simulink model "RefModel_SystemIdentification"  (R2020a)
settings: Solver=ode1  StartTime=0.0  StopTime=inf  FixedStep=Ts_SystemIdentification.Ts_base  MaxStep=Ts  RelTol=1e-3
undefined symbols (not defined in the file or in its folder): SYS_IDENTIFICATION_PARAM
libraries: slctrlblks x4
settings Model: Creator=sl  LastModifiedBy=Administrator
settings DataIOCC: SaveOutput=off  SaveTime=off
settings OptimizationCC: DefaultParameterBehavior=Inlined  EnhancedBackFolding=on  PassReuseOutputArgsAs=Individual arguments  ZeroExternalMemoryAtStartup=off  ZeroInternalMemoryAtStartup=off  OptimizeBlockOrder=speed  DifferentSizesBufferReuse=on  OptimizationCustomize=off  EfficientTunableParamExpr=on
settings DebuggingCC: InheritedTsInSrcMsg=none  ParameterPrecisionLossMsg=none  ParameterTunabilityLossMsg=error  UnconnectedInputMsg=none  UnconnectedOutputMsg=none  UnconnectedLineMsg=none
settings HardwareCC: ProdBitPerPointer=32  ProdBitPerSizeT=32  ProdBitPerPtrDiffT=32  ProdLargestAtomicInteger=Long  ProdLargestAtomicFloat=Double  ProdWordSize=32  ProdHWDeviceType=ARM Compatible->ARM Cortex
settings ModelReferenceCC: ParallelModelReferenceMATLABWorkerInit=Copy Base Workspace  ModelReferenceNumInstancesAllowed=Single
settings SFSimCC: MATLABDynamicMemAlloc=off
settings RTWCC: SystemTargetFile=ert.tlc  GenCodeOnly=on  PackageGeneratedCodeAndArtifacts=on  TemplateMakefile=ert_default_tmf  GenerateReport=on  IncludeHyperlinkInReport=on  LaunchReport=on  GenerateTraceInfo=on  GenerateTraceReport=on  GenerateTraceReportSl=on  GenerateTraceReportSf=on  GenerateTraceReportEml=on
settings CodeAppCC: ForceParamTrailComments=on  IgnoreCustomStorageClasses=off  MaxIdLength=48  OperatorAnnotations=on  SimulinkDataObjDesc=on  SFDataObjDesc=on  MATLABFcnDesc=on  InsertBlockDesc=on  MATLABSourceComments=on
settings ERTTargetCC: TargetLangStandard=C99 (ISO)  GenerateSampleERTMain=on  LogVarNameModifier=none  SupportVariableSizeSignals=on  InlinedParameterPlacement=NonHierarchical  ERTCustomFileTemplate=example_file_process.tlc  ERTFilePackagingFormat=Compact

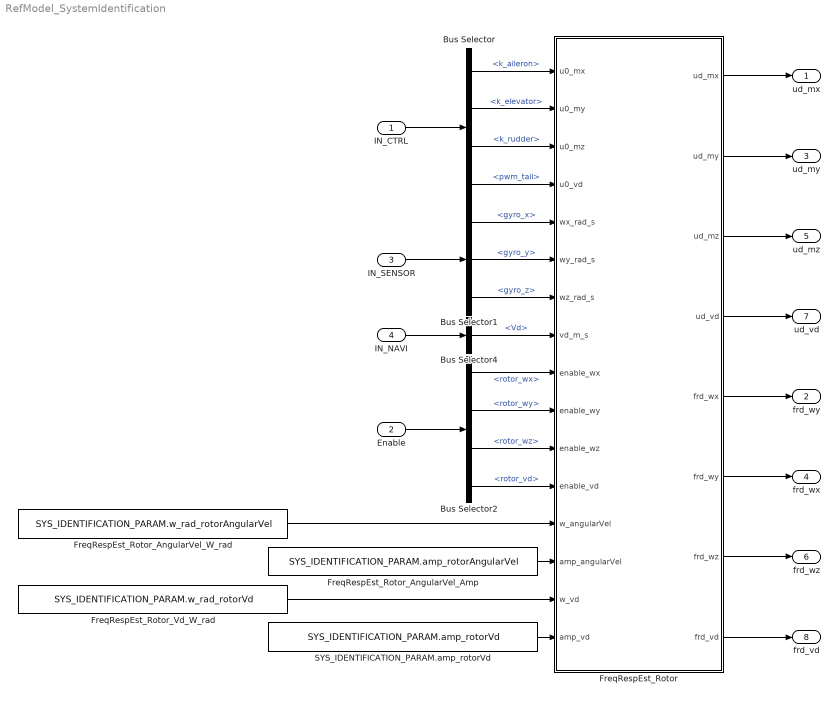
== system RefModel_SystemIdentification ==
  IN_CTRL : Inport  OutDataTypeStr=Bus: BUS_CTRL_Sevro_pwm  PortDimensions=1  BusOutputAsStruct=on
  Enable : Inport  Port=2  OutDataTypeStr=Bus: BUS_SYSIDENTICATION_Enable
  IN_SENSOR : Inport  Port=3  OutDataTypeStr=Bus: BUS_SENSOR  PortDimensions=1  BusOutputAsStruct=on
  IN_NAVI : Inport  Port=4  OutDataTypeStr=Bus: BUS_TO_CONTROL  PortDimensions=1  BusOutputAsStruct=on
  Bus Selector : BusSelector  OutputSignals=k_aileron,k_elevator,k_rudder,pwm_tail
  Bus Selector1 : BusSelector  OutputSignals=IMU1_Control.gyro_x,IMU1_Control.gyro_y,IMU1_Control.gyro_z
  Bus Selector2 : BusSelector  OutputSignals=rotor_wx,rotor_wy,rotor_wz,rotor_vd
  Bus Selector4 : BusSelector  OutputSignals=Vd
  FreqRespEst_Rotor : Subsystem
  FreqRespEst_Rotor_AngularVel_Amp : Constant  Value=SYS_IDENTIFICATION_PARAM.amp_rotorAngularVel
  FreqRespEst_Rotor_AngularVel_W_rad : Constant  Value=SYS_IDENTIFICATION_PARAM.w_rad_rotorAngularVel
  FreqRespEst_Rotor_Vd_W_rad : Constant  Value=SYS_IDENTIFICATION_PARAM.w_rad_rotorVd
  SYS_IDENTIFICATION_PARAM.amp_rotorVd : Constant  Value=SYS_IDENTIFICATION_PARAM.amp_rotorVd
  ud_mx : Outport
  frd_wy : Outport  Port=2
  ud_my : Outport  Port=3
  frd_wx : Outport  Port=4
  ud_mz : Outport  Port=5
  frd_wz : Outport  Port=6
  ud_vd : Outport  Port=7
  frd_vd : Outport  Port=8
  wires:
  Bus Selector2/1 -> FreqRespEst_Rotor/9(enable_wx)  "<rotor_wx>"
  Bus Selector1/2 -> FreqRespEst_Rotor/6(wy_rad_s)  "<gyro_y>"
  FreqRespEst_Rotor/8(frd_vd) -> frd_vd/1
  FreqRespEst_Rotor/4(ud_vd) -> ud_vd/1
  SYS_IDENTIFICATION_PARAM.amp_rotorVd/1 -> FreqRespEst_Rotor/16(amp_vd)
  FreqRespEst_Rotor_AngularVel_W_rad/1 -> FreqRespEst_Rotor/13(w_angularVel)
  FreqRespEst_Rotor_Vd_W_rad/1 -> FreqRespEst_Rotor/15(w_vd)
  FreqRespEst_Rotor/5(frd_wx) -> frd_wy/1
  FreqRespEst_Rotor/2(ud_my) -> ud_my/1
  Bus Selector/4 -> FreqRespEst_Rotor/4(u0_vd)  "<pwm_tail>"
  FreqRespEst_Rotor/3(ud_mz) -> ud_mz/1
  FreqRespEst_Rotor/7(frd_wz) -> frd_wz/1
  FreqRespEst_Rotor/1(ud_mx) -> ud_mx/1
  Bus Selector/3 -> FreqRespEst_Rotor/3(u0_mz)  "<k_rudder>"
  FreqRespEst_Rotor_AngularVel_Amp/1 -> FreqRespEst_Rotor/14(amp_angularVel)
  Bus Selector2/3 -> FreqRespEst_Rotor/11(enable_wz)  "<rotor_wz>"
  Bus Selector2/2 -> FreqRespEst_Rotor/10(enable_wy)  "<rotor_wy>"
  Bus Selector2/4 -> FreqRespEst_Rotor/12(enable_vd)  "<rotor_vd>"
  Bus Selector/2 -> FreqRespEst_Rotor/2(u0_my)  "<k_elevator>"
  Bus Selector1/1 -> FreqRespEst_Rotor/5(wx_rad_s)  "<gyro_x>"
  Bus Selector1/3 -> FreqRespEst_Rotor/7(wz_rad_s)  "<gyro_z>"
  Bus Selector/1 -> FreqRespEst_Rotor/1(u0_mx)  "<k_aileron>"
  FreqRespEst_Rotor/6(frd_wy) -> frd_wx/1
  IN_CTRL/1 -> Bus Selector/1
  IN_SENSOR/1 -> Bus Selector1/1
  IN_NAVI/1 -> Bus Selector4/1
  Bus Selector4/1 -> FreqRespEst_Rotor/8(vd_m_s)  "<Vd>"
  Enable/1 -> Bus Selector2/1

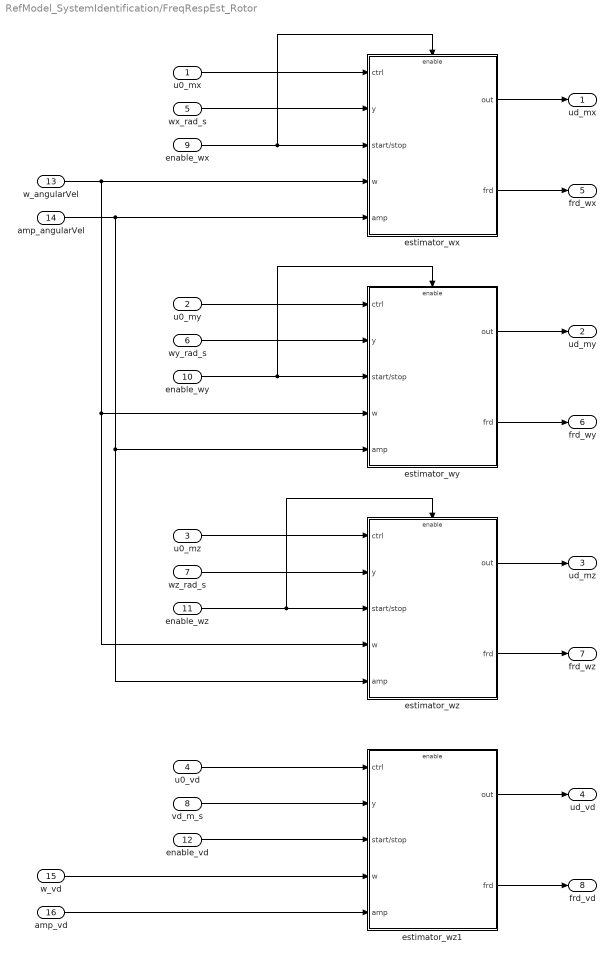
== system RefModel_SystemIdentification/FreqRespEst_Rotor ==
  u0_mx : Inport
  u0_my : Inport  Port=2
  u0_mz : Inport  Port=3
  u0_vd : Inport  Port=4
  wx_rad_s : Inport  Port=5
  wy_rad_s : Inport  Port=6
  wz_rad_s : Inport  Port=7
  vd_m_s : Inport  Port=8
  enable_wx : Inport  Port=9
  enable_wy : Inport  Port=10
  enable_wz : Inport  Port=11
  enable_vd : Inport  Port=12
  w_angularVel : Inport  Port=13
  amp_angularVel : Inport  Port=14
  w_vd : Inport  Port=15
  amp_vd : Inport  Port=16
  estimator_wx : Subsystem
  estimator_wy : Subsystem
  estimator_wz : Subsystem
  estimator_wz1 : Subsystem
  ud_mx : Outport
  ud_my : Outport  Port=2
  ud_mz : Outport  Port=3
  ud_vd : Outport  Port=4
  frd_wx : Outport  Port=5
  frd_wy : Outport  Port=6
  frd_wz : Outport  Port=7
  frd_vd : Outport  Port=8
  wires:
  wz_rad_s/1 -> estimator_wz/2(y)
  estimator_wz/1(out) -> ud_mz/1
  wy_rad_s/1 -> estimator_wy/2(y)
  enable_wz/1 -> estimator_wz/Enable, estimator_wz/3(start/stop)
  estimator_wz/2(frd) -> frd_wz/1
  w_angularVel/1 -> estimator_wx/4(w), estimator_wz/4(w), estimator_wy/4(w)
  vd_m_s/1 -> estimator_wz1/2(y)
  u0_mz/1 -> estimator_wz/1(ctrl)
  estimator_wz1/2(frd) -> frd_vd/1
  amp_vd/1 -> estimator_wz1/5(amp)
  u0_vd/1 -> estimator_wz1/1(ctrl)
  estimator_wz1/1(out) -> ud_vd/1
  estimator_wy/1(out) -> ud_my/1
  enable_vd/1 -> estimator_wz1/3(start/stop)
  enable_wy/1 -> estimator_wy/3(start/stop), estimator_wy/Enable
  estimator_wy/2(frd) -> frd_wy/1
  amp_angularVel/1 -> estimator_wx/5(amp), estimator_wz/5(amp), estimator_wy/5(amp)
  u0_my/1 -> estimator_wy/1(ctrl)
  w_vd/1 -> estimator_wz1/4(w)
  u0_mx/1 -> estimator_wx/1(ctrl)
  wx_rad_s/1 -> estimator_wx/2(y)
  enable_wx/1 -> estimator_wx/Enable, estimator_wx/3(start/stop)
  estimator_wx/1(out) -> ud_mx/1
  estimator_wx/2(frd) -> frd_wx/1

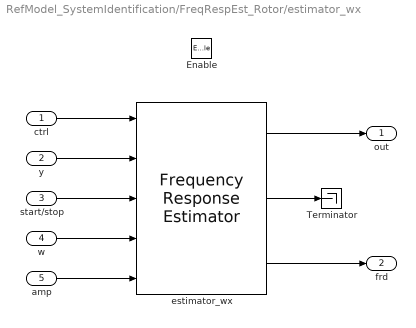
== system RefModel_SystemIdentification/FreqRespEst_Rotor/estimator_wx ==
  ctrl : Inport
  y : Inport  Port=2
  start/stop : Inport  Port=3
  w : Inport  Port=4
  amp : Inport  Port=5
  Enable : EnablePort
  Terminator : Terminator
  estimator_wx : slctrlblks/Frequency Response Estimator  DiscreteTs=Ts_SystemIdentification.Ts_base  OutputMode=control action + perturbation  BlockDataType=double  SineSource=External ports  Frequencies=[0.05 0.1 0.5 1 2 3 4 6 8 10 20 30 40]  FreqUnits=rad/s  Amplitudes=0.05  NumOfFreq=13  ExperimentMode=Sinestream  NumOfSetPeriod=SYS_IDENTIFICATION_PARAM.nSettlingPeriod  NumOfEstPeriod=SYS_IDENTIFICATION_PARAM.nEstimationPeriod  NumOfSlowestPeriod=3  EstimationMode=Online  UseBodePlot=on  BaselinePlant=[]  PlotRefreshFactor=99  BodePlotChoice=VariantBode  ExperimentChoice=VariantSS  OutputChoice=VariantCandD
      settings: SourceProductBaseCode=SD
  out : Outport
  frd : Outport  Port=2
  wires:
  y/1 -> estimator_wx/2
  estimator_wx/2 -> Terminator/1
  estimator_wx/3 -> frd/1
  ctrl/1 -> estimator_wx/1
  amp/1 -> estimator_wx/5
  w/1 -> estimator_wx/4
  estimator_wx/1 -> out/1
  start/stop/1 -> estimator_wx/3

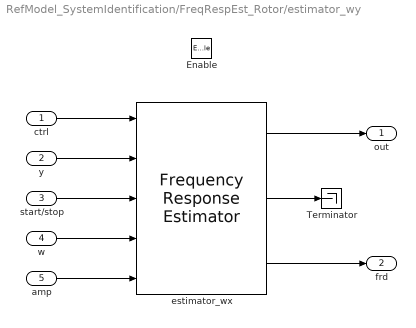
== system RefModel_SystemIdentification/FreqRespEst_Rotor/estimator_wy ==
  ctrl : Inport
  y : Inport  Port=2
  start/stop : Inport  Port=3
  w : Inport  Port=4
  amp : Inport  Port=5
  Enable : EnablePort
  Terminator : Terminator
  estimator_wx : slctrlblks/Frequency Response Estimator  DiscreteTs=Ts_SystemIdentification.Ts_base  OutputMode=control action + perturbation  BlockDataType=double  SineSource=External ports  Frequencies=[0.05 0.1 0.5 1 2 3 4 6 8 10 20 30 40]  FreqUnits=rad/s  Amplitudes=0.05  NumOfFreq=13  ExperimentMode=Sinestream  NumOfSetPeriod=SYS_IDENTIFICATION_PARAM.nSettlingPeriod  NumOfEstPeriod=SYS_IDENTIFICATION_PARAM.nEstimationPeriod  NumOfSlowestPeriod=3  EstimationMode=Online  UseBodePlot=on  BaselinePlant=[]  PlotRefreshFactor=99  BodePlotChoice=VariantBode  ExperimentChoice=VariantSS  OutputChoice=VariantCandD
      settings: SourceProductBaseCode=SD
  out : Outport
  frd : Outport  Port=2
  wires:
  start/stop/1 -> estimator_wx/3
  estimator_wx/1 -> out/1
  w/1 -> estimator_wx/4
  amp/1 -> estimator_wx/5
  ctrl/1 -> estimator_wx/1
  estimator_wx/3 -> frd/1
  estimator_wx/2 -> Terminator/1
  y/1 -> estimator_wx/2

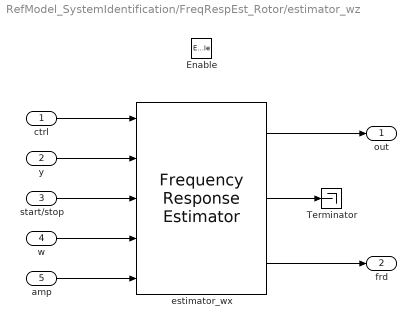
== system RefModel_SystemIdentification/FreqRespEst_Rotor/estimator_wz ==
  ctrl : Inport
  y : Inport  Port=2
  start/stop : Inport  Port=3
  w : Inport  Port=4
  amp : Inport  Port=5
  Enable : EnablePort
  Terminator : Terminator
  estimator_wx : slctrlblks/Frequency Response Estimator  DiscreteTs=Ts_SystemIdentification.Ts_base  OutputMode=control action + perturbation  BlockDataType=double  SineSource=External ports  Frequencies=[0.05 0.1 0.5 1 2 3 4 6 8 10 20 30 40]  FreqUnits=rad/s  Amplitudes=0.05  NumOfFreq=13  ExperimentMode=Sinestream  NumOfSetPeriod=SYS_IDENTIFICATION_PARAM.nSettlingPeriod  NumOfEstPeriod=SYS_IDENTIFICATION_PARAM.nEstimationPeriod  NumOfSlowestPeriod=3  EstimationMode=Online  UseBodePlot=on  BaselinePlant=[]  PlotRefreshFactor=99  BodePlotChoice=VariantBode  ExperimentChoice=VariantSS  OutputChoice=VariantCandD
      settings: SourceProductBaseCode=SD
  out : Outport
  frd : Outport  Port=2
  wires:
  y/1 -> estimator_wx/2
  estimator_wx/2 -> Terminator/1
  estimator_wx/3 -> frd/1
  ctrl/1 -> estimator_wx/1
  amp/1 -> estimator_wx/5
  w/1 -> estimator_wx/4
  estimator_wx/1 -> out/1
  start/stop/1 -> estimator_wx/3

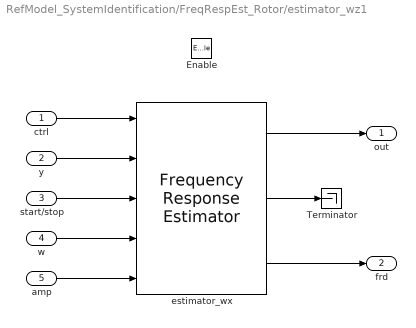
== system RefModel_SystemIdentification/FreqRespEst_Rotor/estimator_wz1 ==
  ctrl : Inport
  y : Inport  Port=2
  start/stop : Inport  Port=3
  w : Inport  Port=4
  amp : Inport  Port=5
  Enable : EnablePort
  Terminator : Terminator
  estimator_wx : slctrlblks/Frequency Response Estimator  DiscreteTs=Ts_SystemIdentification.Ts_base  OutputMode=control action + perturbation  BlockDataType=double  SineSource=External ports  Frequencies=[0.05 0.1 0.5 1 2 3 4 6 8 10 20 30 40]  FreqUnits=rad/s  Amplitudes=0.05  NumOfFreq=13  ExperimentMode=Sinestream  NumOfSetPeriod=SYS_IDENTIFICATION_PARAM.nSettlingPeriod  NumOfEstPeriod=SYS_IDENTIFICATION_PARAM.nEstimationPeriod  NumOfSlowestPeriod=3  EstimationMode=Online  UseBodePlot=on  BaselinePlant=[]  PlotRefreshFactor=99  BodePlotChoice=VariantBode  ExperimentChoice=VariantSS  OutputChoice=VariantCandD
      settings: SourceProductBaseCode=SD
  out : Outport
  frd : Outport  Port=2
  wires:
  start/stop/1 -> estimator_wx/3
  estimator_wx/1 -> out/1
  w/1 -> estimator_wx/4
  amp/1 -> estimator_wx/5
  ctrl/1 -> estimator_wx/1
  estimator_wx/3 -> frd/1
  estimator_wx/2 -> Terminator/1
  y/1 -> estimator_wx/2
